simulink model "Driving_ACC_CACC"  (R2016a)
settings: Solver=ode3  SolverMode=SingleTasking  StartTime=0.0  StopTime=10.0  RelTol=1e-3
undefined symbols (not defined in the file): ACCDelayDistance, Area, ComfortAccelerationParameter, cR, cW, Epsilon, FuelConsumptionFactor, FuelConsumptionOffset, Mass, MaxBreakAcceleration, Power, StandstillDistance, StepTimeCoefficient, TimeGap
settings Model: Creator=Philipp  LastModifiedBy=Schlie
settings DataIOCC: LimitDataPoints=on  SaveFormat=Array
settings OptimizationCC: BlockReduction=off  BooleanDataType=off  ConditionallyExecuteInputs=off  OptimizeBlockIOStorage=off  BufferReuse=off  GlobalBufferReuse=off  ExpressionFolding=off  EnableMemcpy=off  LocalBlockOutputs=off  InitFltsAndDblsToZero=on  EfficientMapNaN2IntZero=off
settings DebuggingCC: SaveWithParameterizedLinksMsg=none  UnderspecifiedInitializationDetection=Classic  MergeDetectMultiDrivingBlocksExec=none  SignalResolutionControl=TryResolveAllWithWarning
settings HardwareCC: ProdBitPerPointer=32  ProdLargestAtomicFloat=None  ProdIntDivRoundTo=Undefined  ProdEndianess=Unspecified  ProdWordSize=32  ProdHWDeviceType=32-bit Generic  TargetBitPerPointer=64  TargetLongLongMode=on  TargetIntDivRoundTo=Zero  TargetEndianess=LittleEndian  TargetWordSize=64  TargetHWDeviceType=MATLAB Host  ProdEqTarget=off
settings ModelReferenceCC: PropagateSignalLabelsOutOfModel=off
settings RTWCC: SystemTargetFile=MESSINA.tlc  TemplateMakefile=MESSINA_Windows_Gnu.tmf  Description=MESSINA Windows GNU Target (API 2)
settings GRTTargetCC: CombineOutputUpdateFcns=off  GRTInterface=on  UseToolchainInfoCompliant=off  RTWCAPISignals=on  RTWCAPIParams=on  RTWCAPIRootIO=on
settings ConfigComp: CovModelRefEnable=Off  CovSFcnEnable=off

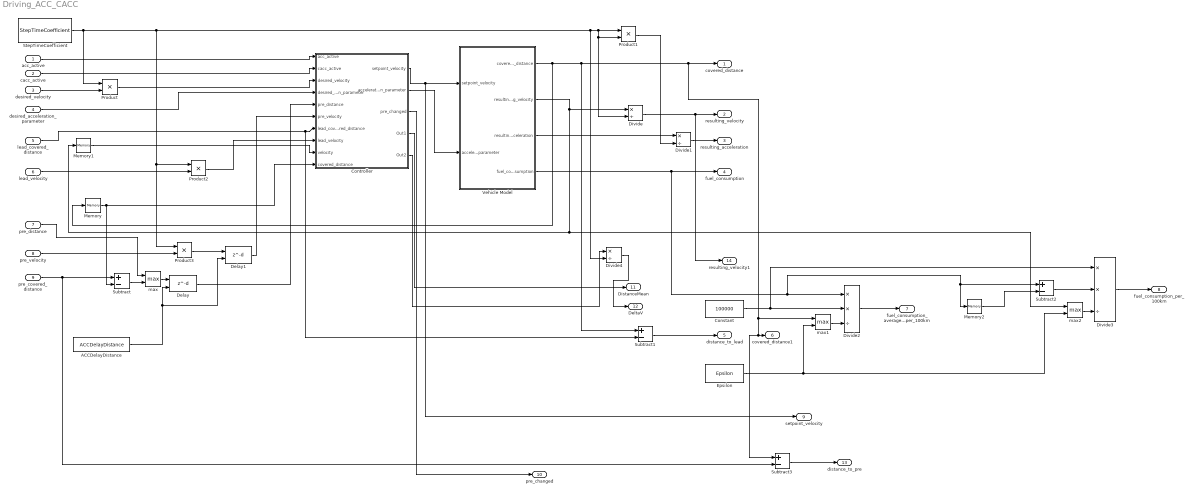
== system Driving_ACC_CACC ==
  acc_active : Inport
  cacc_active : Inport  Port=2
  desired_velocity : Inport  Port=3
  desired_acceleration_parameter : Inport  Port=4
  lead_covered_distance : Inport  Port=5
  lead_velocity : Inport  Port=6
  pre_distance : Inport  Port=7
  pre_velocity : Inport  Port=8
  pre_covered_distance : Inport  Port=9
  ACCDelayDistance : Constant  Value=ACCDelayDistance
  Constant : Constant  Value=100000
  Controller : Subsystem
  Delay : Delay  DelayLengthSource=Input port  DelayLength=ACCDelayDistance
      settings: InputPortMap=u0,p1
  Delay1 : Delay  DelayLengthSource=Input port  DelayLength=ACCDelayDistance
      settings: InputPortMap=u0,p1
  Divide : Product  Inputs=*/
  Divide1 : Product  Inputs=*/
  Divide2 : Product  Inputs=**/
  Divide3 : Product  Inputs=**/
  Divide4 : Product  Inputs=*/
  Epsilon : Constant  Value=Epsilon
  Memory : Memory
  Memory1 : Memory
  Memory2 : Memory
  Product{,1..3} (4 alike) : Product
  StepTimeCoefficient : Constant  Value=StepTimeCoefficient
  Subtract{,1..3} (4 alike) : Sum  Inputs=+-
  Vehicle Model : Subsystem
  max : MinMax  Function=max  Inputs=2
  max1 : MinMax  Function=max  Inputs=2
  max2 : MinMax  Function=max  Inputs=2
  covered_distance : Outport
  resulting_velocity : Outport  Port=2
  resulting_acceleration : Outport  Port=3
  fuel_consumption : Outport  Port=4
  distance_to_lead : Outport  Port=5
  covered_distance1 : Outport  Port=6
  fuel_consumption_average_per_100km : Outport  Port=7
  fuel_consumption_per_100km : Outport  Port=8
  setpoint_velocity : Outport  Port=9
  pre_changed : Outport  Port=10
  DistanceMean : Outport  Port=11
  DeltaV : Outport  Port=12
  distance_to_pre : Outport  Port=13
  resulting_velocity1 : Outport  Port=14
  wires:
  Vehicle Model/3(resulting_acceleration) -> Divide1/1
  cacc_active/1 -> Controller/2(cacc_active)
  Product/1 -> Controller/3(desired_velocity)
  pre_distance/1 -> max/1
  lead_covered_distance/1 -> Subtract1/2, Controller/7(lead_covered_distance)
  Vehicle Model/2(resulting_velocity) -> Divide/1, Memory1/1, max2/1
  Vehicle Model/1(covered_distance) -> Memory/1, Subtract1/1, Subtract3/1, covered_distance1/1, max1/1, covered_distance/1
  Memory/1 -> Controller/10(covered_distance), Subtract/2
  Memory1/1 -> Controller/9(velocity)
  acc_active/1 -> Controller/1(acc_active)
  desired_velocity/1 -> Product/2
  Divide/1 -> resulting_velocity1/1, resulting_velocity/1
  Divide1/1 -> resulting_acceleration/1
  Product1/1 -> Divide1/2
  desired_acceleration_parameter/1 -> Controller/4(desired_acceleration_parameter)
  pre_covered_distance/1 -> Subtract/1, Subtract3/2
  max/1 -> Delay/1
  Subtract/1 -> max/2
  Subtract1/1 -> distance_to_lead/1
  Controller/1(setpoint_velocity) -> setpoint_velocity/1, Vehicle Model/1(setpoint_velocity)
  Controller/2(acceleration_parameter) -> Vehicle Model/2(acceleration_parameter)
  Vehicle Model/4(fuel_consumption) -> Memory2/1, Subtract2/1, Divide2/1, fuel_consumption/1
  Constant/1 -> Divide3/1, Divide2/2
  Divide2/1 -> fuel_consumption_average_per_100km/1
  Memory2/1 -> Subtract2/2
  Subtract2/1 -> Divide3/2
  Divide3/1 -> fuel_consumption_per_100km/1
  max1/1 -> Divide2/3
  max2/1 -> Divide3/3
  Epsilon/1 -> max2/2, max1/2
  Delay/1 -> Controller/5(pre_distance)
  ACCDelayDistance/1 -> Delay/2, Delay1/2
  Controller/3(pre_changed) -> pre_changed/1
  Controller/5(Out2) -> Divide4/1
  StepTimeCoefficient/1 -> Product3/1, Product2/1, Divide4/2, Product1/1, Product1/2, Divide/2, Product/1
  Controller/4(Out1) -> DistanceMean/1
  Divide4/1 -> DeltaV/1
  Subtract3/1 -> distance_to_pre/1
  pre_velocity/1 -> Product3/2
  lead_velocity/1 -> Product2/2
  Product2/1 -> Controller/8(lead_velocity)
  Product3/1 -> Delay1/1
  Delay1/1 -> Controller/6(pre_velocity)

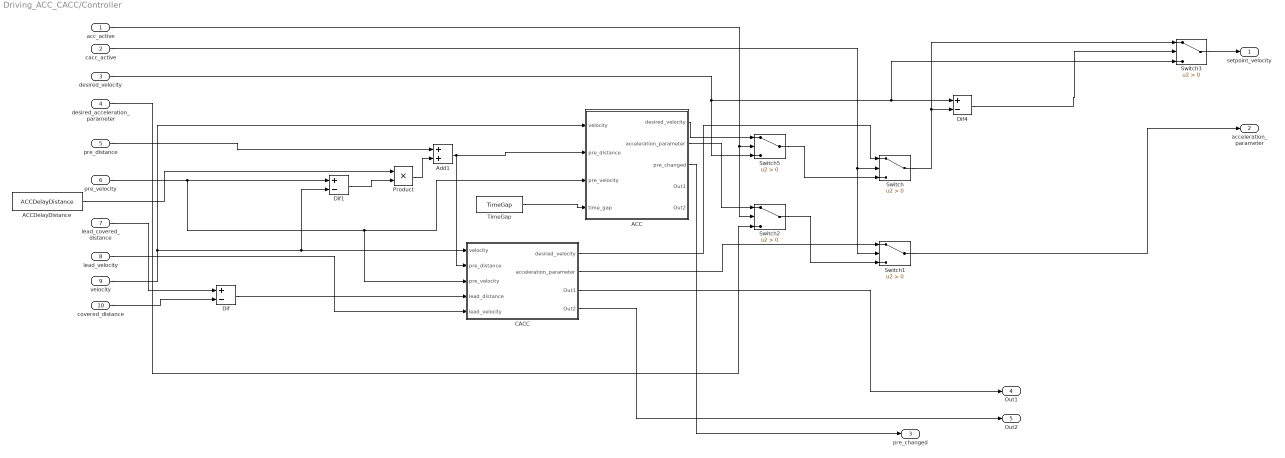
== system Driving_ACC_CACC/Controller ==
  acc_active : Inport
  cacc_active : Inport  Port=2
  desired_velocity : Inport  Port=3
  desired_acceleration_parameter : Inport  Port=4
  pre_distance : Inport  Port=5
  pre_velocity : Inport  Port=6
  lead_covered_distance : Inport  Port=7
  lead_velocity : Inport  Port=8
  velocity : Inport  Port=9
  covered_distance : Inport  Port=10
  ACC : Subsystem
  ACCDelayDistance : Constant  Value=ACCDelayDistance
  Add1 : Sum
  CACC : Subsystem
  Dif : Sum  Inputs=+-
  Dif1 : Sum  Inputs=+-
  Dif4 : Sum  Inputs=+-
  Product : Product
  Switch{,1..3,5} (5 alike) : Switch  Criteria=u2 > Threshold
  TimeGap : Constant  Value=TimeGap
  setpoint_velocity : Outport
  acceleration_parameter : Outport  Port=2
  pre_changed : Outport  Port=3
  Out1 : Outport  Port=4
  Out2 : Outport  Port=5
  wires:
  velocity/1 -> ACC/1(velocity), Dif1/2, CACC/1(velocity)
  lead_covered_distance/1 -> Dif/1
  covered_distance/1 -> Dif/2
  Dif/1 -> CACC/4(lead_distance)
  Switch3/1 -> setpoint_velocity/1
  desired_velocity/1 -> Switch5/3, Switch3/3, Dif4/1
  Switch1/1 -> acceleration_parameter/1
  desired_acceleration_parameter/1 -> Switch2/3
  pre_distance/1 -> Add1/1
  Switch/1 -> Switch3/1, Dif4/2
  Dif4/1 -> Switch3/2
  cacc_active/1 -> Switch1/2, Switch/2
  CACC/1(desired_velocity) -> Switch/1
  CACC/2(acceleration_parameter) -> Switch1/1
  Switch2/1 -> Switch1/3
  Switch5/1 -> Switch/3
  acc_active/1 -> Switch2/2, Switch5/2
  ACC/2(acceleration_parameter) -> Switch2/1
  ACC/1(desired_velocity) -> Switch5/1
  ACCDelayDistance/1 -> Product/1
  TimeGap/1 -> ACC/4(time_gap)
  Add1/1 -> ACC/2(pre_distance), CACC/2(pre_distance)
  Product/1 -> Add1/2
  ACC/3(pre_changed) -> pre_changed/1
  CACC/3(Out1) -> Out1/1
  CACC/4(Out2) -> Out2/1
  lead_velocity/1 -> CACC/5(lead_velocity)
  pre_velocity/1 -> ACC/3(pre_velocity), CACC/3(pre_velocity), Dif1/1
  Dif1/1 -> Product/2

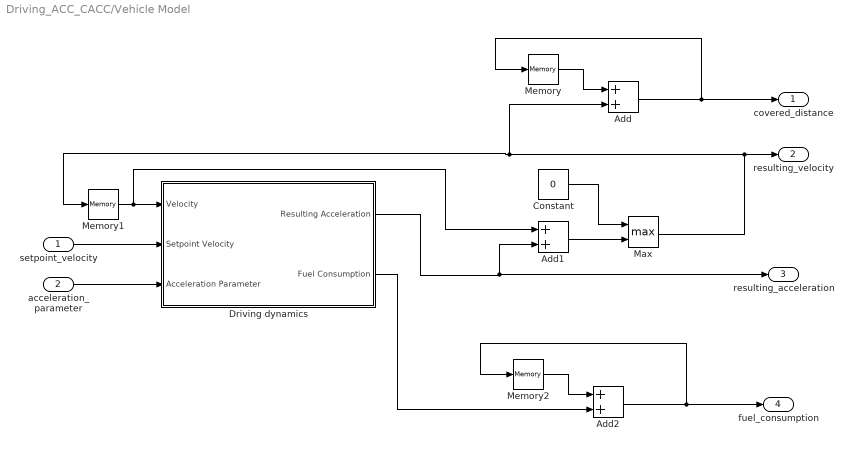
== system Driving_ACC_CACC/Vehicle Model ==
  setpoint_velocity : Inport
  acceleration_parameter : Inport  Port=2
  Add : Sum
  Add1 : Sum
  Add2 : Sum
  Constant : Constant  Value=0
  Driving dynamics : Subsystem
  Max : MinMax  Function=max  Inputs=2
  Memory : Memory
  Memory1 : Memory
  Memory2 : Memory
  covered_distance : Outport
  resulting_velocity : Outport  Port=2
  resulting_acceleration : Outport  Port=3
  fuel_consumption : Outport  Port=4
  wires:
  Add/1 -> Memory/1, covered_distance/1
  Max/1 -> Memory1/1, Add/2, resulting_velocity/1
  setpoint_velocity/1 -> Driving dynamics/2(Setpoint Velocity)
  acceleration_parameter/1 -> Driving dynamics/3(Acceleration Parameter)
  Memory1/1 -> Add1/1, Driving dynamics/1(Velocity)
  Memory/1 -> Add/1
  Driving dynamics/1(Resulting Acceleration) -> Add1/2, resulting_acceleration/1
  Add1/1 -> Max/2
  Constant/1 -> Max/1
  Add2/1 -> Memory2/1, fuel_consumption/1
  Driving dynamics/2(Fuel Consumption) -> Add2/2
  Memory2/1 -> Add2/1

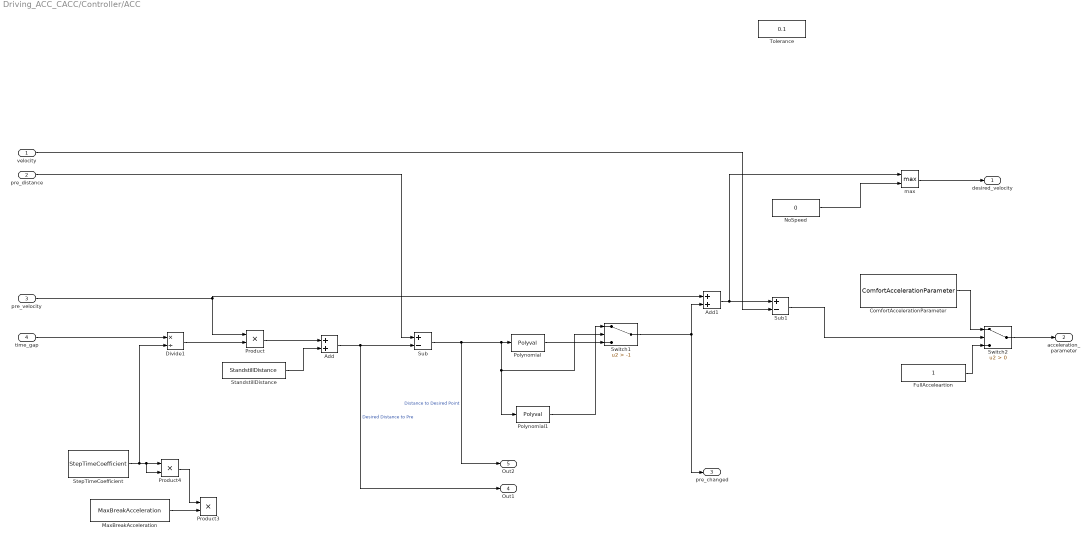
== system Driving_ACC_CACC/Controller/ACC ==
  velocity : Inport
  pre_distance : Inport  Port=2
  pre_velocity : Inport  Port=3
  time_gap : Inport  Port=4
  Add : Sum
  Add1 : Sum
  ComfortAccelerationParameter : Constant  Value=ComfortAccelerationParameter
  Divide1 : Product  Inputs=*/
  FullAcceleartion : Constant
  MaxBreakAcceleration : Constant  Value=MaxBreakAcceleration
  NoSpeed : Constant  Value=0
  Polynomial : Polyval  Coefs=[0.002, 0, 0, 0]
  Polynomial1 : Polyval  Coefs=[0.002,0]
  Product : Product
  Product3 : Product
  Product4 : Product
  StandstillDistance : Constant  Value=StandstillDistance
  StepTimeCoefficient : Constant  Value=StepTimeCoefficient
  Sub : Sum  Inputs=+-
  Sub1 : Sum  Inputs=+-
  Switch1 : Switch  Criteria=u2 > Threshold  Threshold=-1
  Switch2 : Switch  Criteria=u2 > Threshold
  Tolerance : Constant  Value=0.1
  max : MinMax  Function=max  Inputs=2
  desired_velocity : Outport
  acceleration_parameter : Outport  Port=2
  pre_changed : Outport  Port=3
  Out1 : Outport  Port=4
  Out2 : Outport  Port=5
  wires:
  pre_distance/1 -> Sub/1
  max/1 -> desired_velocity/1
  Switch2/1 -> acceleration_parameter/1
  FullAcceleartion/1 -> Switch2/3
  StepTimeCoefficient/1 -> Divide1/2, Product4/1, Product4/2
  MaxBreakAcceleration/1 -> Product3/2
  Product4/1 -> Product3/1
  NoSpeed/1 -> max/2
  time_gap/1 -> Divide1/1
  ComfortAccelerationParameter/1 -> Switch2/1
  pre_velocity/1 -> Add1/1, Product/1
  Divide1/1 -> Product/2
  Product/1 -> Add/1
  StandstillDistance/1 -> Add/2
  Add/1 -> Out1/1, Sub/2  "Desired Distance to Pre"
  Sub/1 -> Out2/1, Polynomial1/1, Switch1/2, Polynomial/1  "Distance to Desired Point"
  Add1/1 -> Sub1/1, max/1
  velocity/1 -> Sub1/2
  Sub1/1 -> Switch2/2
  Polynomial/1 -> Switch1/3
  Polynomial1/1 -> Switch1/1
  Switch1/1 -> Add1/2, pre_changed/1

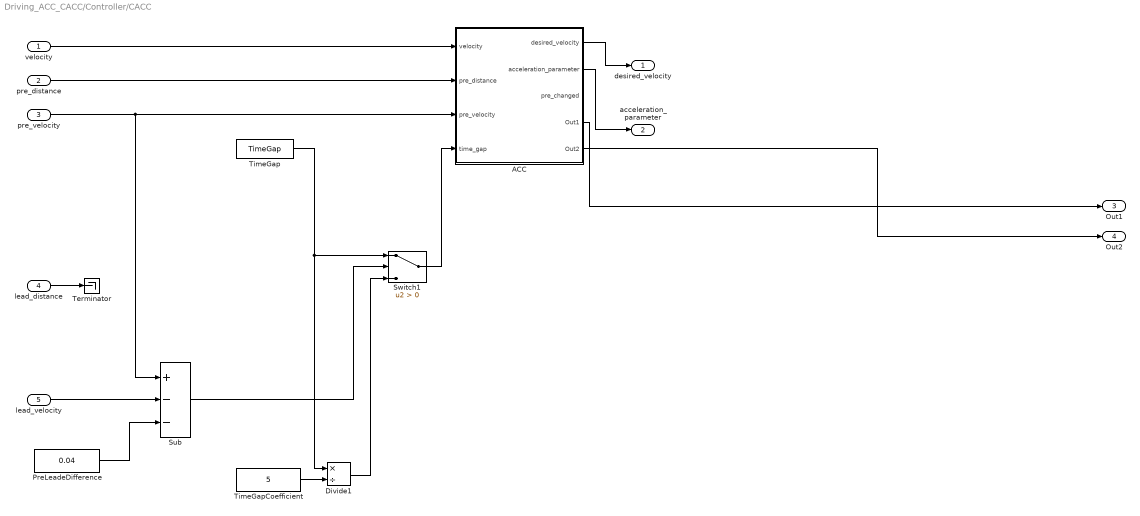
== system Driving_ACC_CACC/Controller/CACC ==
  velocity : Inport
  pre_distance : Inport  Port=2
  pre_velocity : Inport  Port=3
  lead_distance : Inport  Port=4
  lead_velocity : Inport  Port=5
  ACC : Subsystem
  Divide1 : Product  Inputs=*/
  PreLeadeDifference : Constant  Value=0.04
  Sub : Sum  Inputs=+--
  Switch1 : Switch  Criteria=u2 > Threshold
  Terminator : Terminator
  TimeGap : Constant  Value=TimeGap
  TimeGapCoefficient : Constant  Value=5
  desired_velocity : Outport
  acceleration_parameter : Outport  Port=2
  Out1 : Outport  Port=3
  Out2 : Outport  Port=4
  wires:
  velocity/1 -> ACC/1(velocity)
  pre_distance/1 -> ACC/2(pre_distance)
  pre_velocity/1 -> Sub/1, ACC/3(pre_velocity)
  lead_velocity/1 -> Sub/2
  TimeGap/1 -> Divide1/1, Switch1/1
  lead_distance/1 -> Terminator/1
  ACC/1(desired_velocity) -> desired_velocity/1
  ACC/2(acceleration_parameter) -> acceleration_parameter/1
  ACC/4(Out1) -> Out1/1
  ACC/5(Out2) -> Out2/1
  Switch1/1 -> ACC/4(time_gap)
  Sub/1 -> Switch1/2
  PreLeadeDifference/1 -> Sub/3
  TimeGapCoefficient/1 -> Divide1/2
  Divide1/1 -> Switch1/3

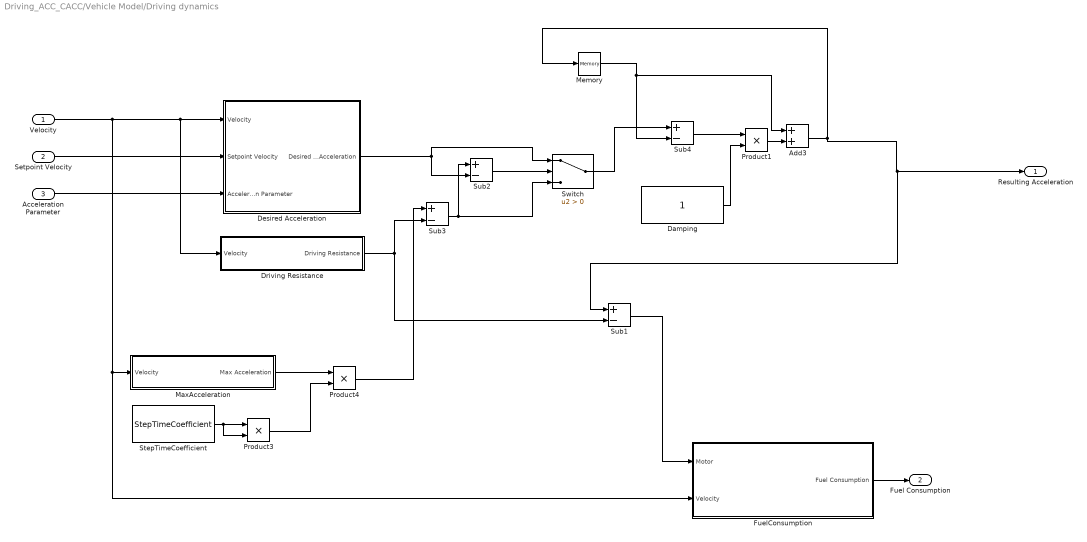
== system Driving_ACC_CACC/Vehicle Model/Driving dynamics ==
  Velocity : Inport
  Setpoint Velocity : Inport  Port=2
  Acceleration Parameter : Inport  Port=3
  Add3 : Sum
  Damping : Constant
  Desired Acceleration : Subsystem
  Driving Resistance : Subsystem
  FuelConsumption : Subsystem
  MaxAcceleration : Subsystem
  Memory : Memory
  Product1 : Product
  Product3 : Product
  Product4 : Product
  StepTimeCoefficient : Constant  Value=StepTimeCoefficient
  Sub{1..4} (4 alike) : Sum  Inputs=+-
  Switch : Switch  Criteria=u2 > Threshold
  Resulting Acceleration : Outport
  Fuel Consumption : Outport  Port=2
  wires:
  Setpoint Velocity/1 -> Desired Acceleration/2(Setpoint Velocity)
  Acceleration Parameter/1 -> Desired Acceleration/3(Acceleration Parameter)
  StepTimeCoefficient/1 -> Product3/1, Product3/2
  MaxAcceleration/1(Max Acceleration) -> Product4/1
  Product3/1 -> Product4/2
  Product4/1 -> Sub3/1
  Velocity/1 -> FuelConsumption/2(Velocity), MaxAcceleration/1(Velocity), Driving Resistance/1(Velocity), Desired Acceleration/1(Velocity)
  FuelConsumption/1(Fuel Consumption) -> Fuel Consumption/1
  Driving Resistance/1(Driving Resistance) -> Sub3/2, Sub1/2
  Sub2/1 -> Switch/2
  Sub3/1 -> Switch/3, Sub2/1
  Desired Acceleration/1(Desired Acceleration) -> Sub2/2, Switch/1
  Sub1/1 -> FuelConsumption/1(Motor)
  Memory/1 -> Add3/1, Sub4/2
  Switch/1 -> Sub4/1
  Sub4/1 -> Product1/1
  Damping/1 -> Product1/2
  Add3/1 -> Sub1/1, Resulting Acceleration/1, Memory/1
  Product1/1 -> Add3/2

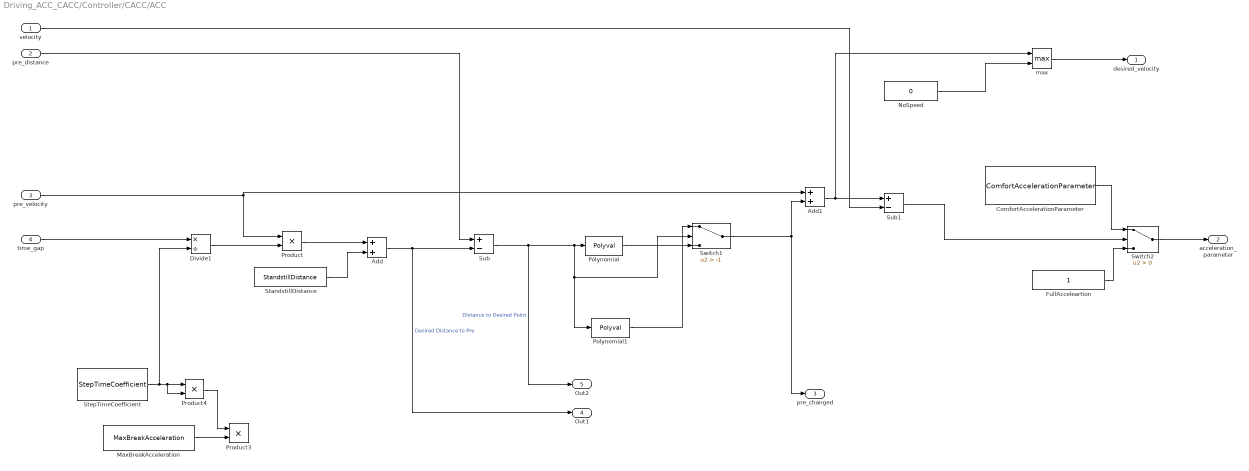
== system Driving_ACC_CACC/Controller/CACC/ACC ==
  velocity : Inport
  pre_distance : Inport  Port=2
  pre_velocity : Inport  Port=3
  time_gap : Inport  Port=4
  Add : Sum
  Add1 : Sum
  ComfortAccelerationParameter : Constant  Value=ComfortAccelerationParameter
  Divide1 : Product  Inputs=*/
  FullAcceleartion : Constant
  MaxBreakAcceleration : Constant  Value=MaxBreakAcceleration
  NoSpeed : Constant  Value=0
  Polynomial : Polyval  Coefs=[0.002, 0, 0, 0]
  Polynomial1 : Polyval  Coefs=[0.002,0]
  Product : Product
  Product3 : Product
  Product4 : Product
  StandstillDistance : Constant  Value=StandstillDistance
  StepTimeCoefficient : Constant  Value=StepTimeCoefficient
  Sub : Sum  Inputs=+-
  Sub1 : Sum  Inputs=+-
  Switch1 : Switch  Criteria=u2 > Threshold  Threshold=-1
  Switch2 : Switch  Criteria=u2 > Threshold
  max : MinMax  Function=max  Inputs=2
  desired_velocity : Outport
  acceleration_parameter : Outport  Port=2
  pre_changed : Outport  Port=3
  Out1 : Outport  Port=4
  Out2 : Outport  Port=5
  wires:
  pre_distance/1 -> Sub/1
  max/1 -> desired_velocity/1
  Switch2/1 -> acceleration_parameter/1
  FullAcceleartion/1 -> Switch2/3
  StepTimeCoefficient/1 -> Divide1/2, Product4/1, Product4/2
  MaxBreakAcceleration/1 -> Product3/2
  Product4/1 -> Product3/1
  NoSpeed/1 -> max/2
  time_gap/1 -> Divide1/1
  ComfortAccelerationParameter/1 -> Switch2/1
  pre_velocity/1 -> Add1/1, Product/1
  Divide1/1 -> Product/2
  Product/1 -> Add/1
  StandstillDistance/1 -> Add/2
  Add/1 -> Out1/1, Sub/2  "Desired Distance to Pre"
  Sub/1 -> Out2/1, Polynomial1/1, Switch1/2, Polynomial/1  "Distance to Desired Point"
  Add1/1 -> Sub1/1, max/1
  velocity/1 -> Sub1/2
  Sub1/1 -> Switch2/2
  Polynomial/1 -> Switch1/3
  Polynomial1/1 -> Switch1/1
  Switch1/1 -> Add1/2, pre_changed/1

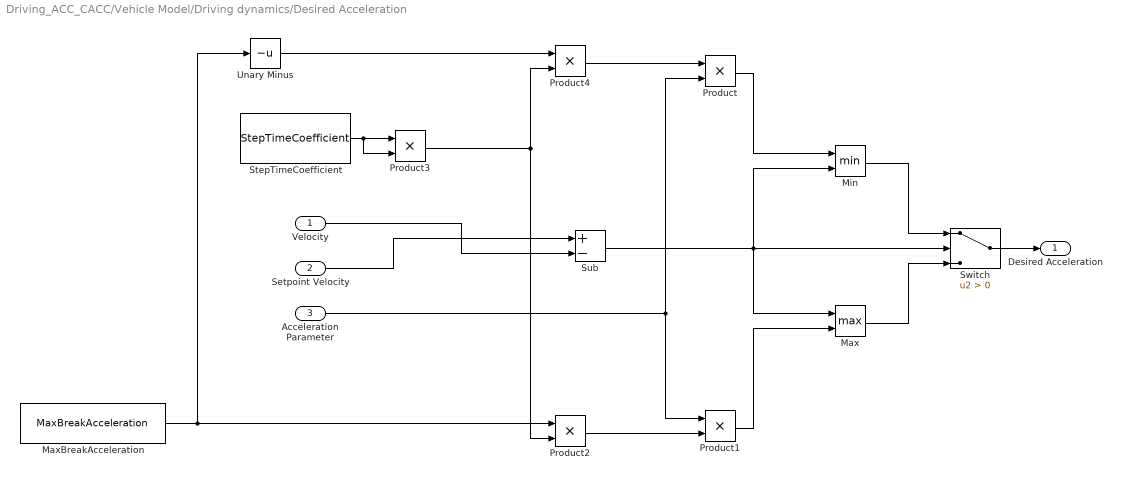
== system Driving_ACC_CACC/Vehicle Model/Driving dynamics/Desired Acceleration ==
  Velocity : Inport
  Setpoint Velocity : Inport  Port=2
  Acceleration Parameter : Inport  Port=3
  Max : MinMax  Function=max  Inputs=2
  MaxBreakAcceleration : Constant  Value=MaxBreakAcceleration
  Min : MinMax  Inputs=2
  Product{,1..4} (5 alike) : Product
  StepTimeCoefficient : Constant  Value=StepTimeCoefficient
  Sub : Sum  Inputs=+-
  Switch : Switch  Criteria=u2 > Threshold
  Unary Minus : UnaryMinus
  Desired Acceleration : Outport
  wires:
  Sub/1 -> Min/2, Max/1, Switch/2
  Velocity/1 -> Sub/2
  Setpoint Velocity/1 -> Sub/1
  Acceleration Parameter/1 -> Product/2, Product1/1
  Product/1 -> Min/1
  Product1/1 -> Max/2
  StepTimeCoefficient/1 -> Product3/1, Product3/2
  Product2/1 -> Product1/2
  Unary Minus/1 -> Product4/1
  Product3/1 -> Product2/2, Product4/2
  Product4/1 -> Product/1
  Max/1 -> Switch/3
  Min/1 -> Switch/1
  MaxBreakAcceleration/1 -> Unary Minus/1, Product2/1
  Switch/1 -> Desired Acceleration/1

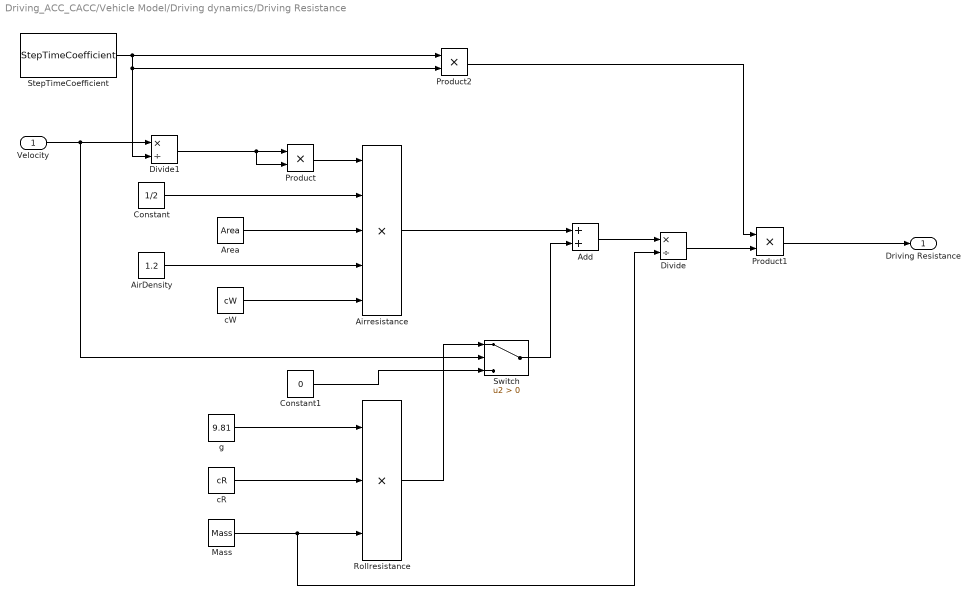
== system Driving_ACC_CACC/Vehicle Model/Driving dynamics/Driving Resistance ==
  Velocity : Inport
  Add : Sum
  AirDensity : Constant  Value=1.2
  Airresistance : Product  Inputs=5
  Area : Constant  Value=Area
  Constant : Constant  Value=1/2
  "Constant1 " : Constant  Value=0
  Divide : Product  Inputs=*/
  Divide1 : Product  Inputs=*/
  Mass : Constant  Value=Mass
  Product : Product
  Product1 : Product
  Product2 : Product
  Rollresistance : Product  Inputs=3
  StepTimeCoefficient : Constant  Value=StepTimeCoefficient
  Switch : Switch  Criteria=u2 > Threshold
  cR : Constant  Value=cR
  cW : Constant  Value=cW
  g : Constant  Value=9.81
  Driving Resistance : Outport
  wires:
  Divide1/1 -> Product/2, Product/1
  g/1 -> Rollresistance/1
  cR/1 -> Rollresistance/2
  Mass/1 -> Divide/2, Rollresistance/3
  cW/1 -> Airresistance/5
  AirDensity/1 -> Airresistance/4
  Area/1 -> Airresistance/3
  Constant/1 -> Airresistance/2
  Product/1 -> Airresistance/1
  Airresistance/1 -> Add/1
  Rollresistance/1 -> Switch/1
  Add/1 -> Divide/1
  Product1/1 -> Driving Resistance/1
  StepTimeCoefficient/1 -> Product2/1, Divide1/2, Product2/2
  Velocity/1 -> Switch/2, Divide1/1
  Divide/1 -> Product1/2
  Product2/1 -> Product1/1
  Switch/1 -> Add/2
  "Constant1 "/1 -> Switch/3

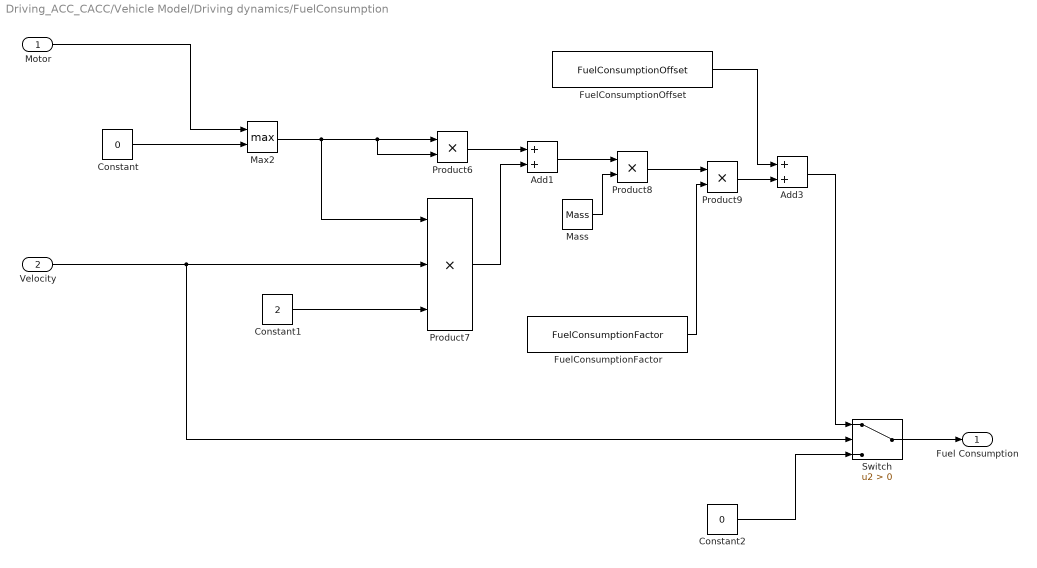
== system Driving_ACC_CACC/Vehicle Model/Driving dynamics/FuelConsumption ==
  Motor : Inport
  Velocity : Inport  Port=2
  Add1 : Sum
  Add3 : Sum
  Constant : Constant  Value=0
  Constant1 : Constant  Value=2
  Constant2 : Constant  Value=0
  FuelConsumptionFactor : Constant  Value=FuelConsumptionFactor
  FuelConsumptionOffset : Constant  Value=FuelConsumptionOffset
  Mass : Constant  Value=Mass
  Max2 : MinMax  Function=max  Inputs=2
  Product6 : Product
  Product7 : Product  Inputs=3
  Product8 : Product
  Product9 : Product
  Switch : Switch  Criteria=u2 > Threshold
  Fuel Consumption : Outport
  wires:
  Constant/1 -> Max2/2
  Max2/1 -> Product7/1, Product6/2, Product6/1
  Constant1/1 -> Product7/3
  Product6/1 -> Add1/1
  Product7/1 -> Add1/2
  Add1/1 -> Product8/1
  Mass/1 -> Product8/2
  Product8/1 -> Product9/1
  FuelConsumptionFactor/1 -> Product9/2
  Product9/1 -> Add3/2
  FuelConsumptionOffset/1 -> Add3/1
  Add3/1 -> Switch/1
  Velocity/1 -> Switch/2, Product7/2
  Motor/1 -> Max2/1
  Switch/1 -> Fuel Consumption/1
  Constant2/1 -> Switch/3

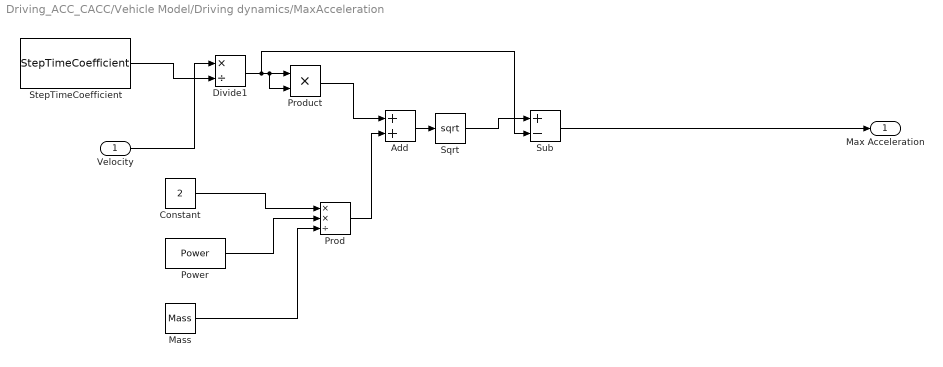
== system Driving_ACC_CACC/Vehicle Model/Driving dynamics/MaxAcceleration ==
  Velocity : Inport
  Add : Sum
  Constant : Constant  Value=2
  Divide1 : Product  Inputs=*/
  Mass : Constant  Value=Mass
  Power : Constant  Value=Power
  Prod : Product  Inputs=**/
  Product : Product
  Sqrt : Sqrt  SaturateOnIntegerOverflow=on
  StepTimeCoefficient : Constant  Value=StepTimeCoefficient
  Sub : Sum  Inputs=+-
  Max Acceleration : Outport
  wires:
  StepTimeCoefficient/1 -> Divide1/2
  Velocity/1 -> Divide1/1
  Sub/1 -> Max Acceleration/1
  Divide1/1 -> Sub/2, Product/2, Product/1
  Constant/1 -> Prod/1
  Power/1 -> Prod/2
  Mass/1 -> Prod/3
  Product/1 -> Add/1
  Prod/1 -> Add/2
  Add/1 -> Sqrt/1
  Sqrt/1 -> Sub/1
